simulink model "BrowarModel"  (R2024a)
settings: Solver=ode5  StartTime=0.0  StopTime=inf  FixedStep=0.1  RelTol=1e-3
undefined symbols (not defined in the file or in its folder): localhost, Matrikon, OI
libraries: opclib x24
(part 7 of 9)

== system BrowarModel/System dozowania drozdzy/System dozowania drozdzy/Zawor trojdrozny ==
  note: Zawor trojdrozny
  Sterowanie rusztem : Inport
  Przeplyw zasilanie : Inport  Port=2
  Dot Product : DotProduct  OutDataTypeStr=Inherit: Inherit via internal rule
  Relay : Relay  OffOutputValue=-1
  Transfer Fcn : TransferFcn  Denominator=[0.1 1]
  Przeplyw sterowanie : Outport
  wires:
  Transfer Fcn/1 -> Przeplyw sterowanie/1
  Dot Product/1 -> Transfer Fcn/1
  Przeplyw zasilanie/1 -> Dot Product/1
  Relay/1 -> Dot Product/2
  Sterowanie rusztem/1 -> Relay/1

== system BrowarModel/System dozowania drozdzy/WT805/Zaklocenia pomiarowe ==
  Product1 : Product  InputSameDT=on  RndMeth=Zero  SaturateOnIntegerOverflow=on  OutDataTypeStr=Inherit: Same as first input
  Product3 : Product  InputSameDT=on  RndMeth=Zero  SaturateOnIntegerOverflow=on  OutDataTypeStr=Inherit: Same as first input
  Random Number : RandomNumber  Variance=.04  Seed=4365624  SampleTime=0.1
  Transfer Fcn1 : TransferFcn  Denominator=[0.5 1]
  Transfer Fcn2 : TransferFcn  Denominator=[0.5 1]
  Zaklocenia pomiarowe : Constant  Value=ZakloceniaPom
  Out : Outport
  wires:
  Random Number/1 -> Product3/1
  Product3/1 -> Transfer Fcn1/1
  Transfer Fcn1/1 -> Transfer Fcn2/1
  Transfer Fcn2/1 -> Out/1
  Zaklocenia pomiarowe/1 -> Product1/2
  [ZaklPom] -> Product1/1
  Product1/1 -> Product3/2

== system BrowarModel/System dozowania drozdzy/XT804/Zaklocenia pomiarowe ==
  Product1 : Product  InputSameDT=on  RndMeth=Zero  SaturateOnIntegerOverflow=on  OutDataTypeStr=Inherit: Same as first input
  Product3 : Product  InputSameDT=on  RndMeth=Zero  SaturateOnIntegerOverflow=on  OutDataTypeStr=Inherit: Same as first input
  Random Number : RandomNumber  Variance=.5  Seed=4365624  SampleTime=0.1
  Transfer Fcn1 : TransferFcn  Denominator=[0.5 1]
  Transfer Fcn2 : TransferFcn  Denominator=[0.5 1]
  Zaklocenia pomiarowe : Constant  Value=ZakloceniaPom
  Out : Outport
  wires:
  Random Number/1 -> Product3/1
  Product3/1 -> Transfer Fcn1/1
  Transfer Fcn1/1 -> Transfer Fcn2/1
  Transfer Fcn2/1 -> Out/1
  Zaklocenia pomiarowe/1 -> Product1/2
  [ZaklPom] -> Product1/1
  Product1/1 -> Product3/2

== system BrowarModel/Kadz fermentacyjna/Kadz fermentacyjna/Kadz/Model akumulacji ciepla w zbiorniku z ciecza ==
  Objetosc cieczy w zbiorniku : Inport
  Strumien odplywu cieczy : Inport  Port=2
  Strumien doplywu cieczy : Inport  Port=3
  Strumien cieplna dostepny : Inport  Port=4
  Strumien cieplo traconego : Inport  Port=5
  Temperatura strumien doplywu cieczy : Inport  Port=6
  1/gestosc cieczy : Gain  Gain=1/1000
  Cieplo : Integrator  LimitOutput=on  LowerSaturationLimit=0
  Cieplo parowania : Constant  Value=2257000
  Cieplo strumienia cieczy doplywajacej : Subsystem
  Cieplo strumienia cieczy odplywajacej : Subsystem
  "Cieplo wlasciwe " : Constant  Value=4189.9
  Divide : Product  Inputs=/*
  Divide1 : Product  Inputs=*/
  Divide2 : Product  Inputs=*/
  "Dot " : DotProduct  OutDataTypeStr=Inherit: Inherit via internal rule
  Dot 1 : DotProduct  OutDataTypeStr=Inherit: Inherit via internal rule
  Gestosc cieczy : Gain  Gain=1000
  Saturation : Saturate  UpperLimit=inf  LowerLimit=0
  Sum{1..2,4..5} (4 alike) : Sum  Inputs=|+-
  Sum10 : Sum  Inputs=|++
  Sum3 : Sum  Inputs=|-+
  Sum7 : Sum  Inputs=|++
  Temperatura parowania : Constant  Value=100
  Zamiana C->K : Constant  Value=273.6
  Srumien cieczy odparowanej : Outport
  Srednia temperaturacie czy : Outport  Port=2
  Strumien ciepla odebrany : Outport  Port=3
  wires:
  Strumien cieplna dostepny/1 -> Strumien ciepla odebrany/1, Sum10/2  "J/s"
  Sum5/1 -> Sum4/1, Srednia temperaturacie czy/1
  Strumien doplywu cieczy/1 -> Cieplo strumienia cieczy doplywajacej/2(Strumien cieczy)  "m3/s"
  Zamiana C->K/1 -> Sum5/2
  "Cieplo wlasciwe "/1 -> Divide1/2, Dot 1/2  "J/(kg*K)"
  Cieplo strumienia cieczy doplywajacej/1(Strumien ciepla) -> Sum3/2  "J/s"
  Temperatura strumien doplywu cieczy/1 -> Cieplo strumienia cieczy doplywajacej/1(Temperatura strumienia cieczy)  "dec C"
  Divide1/1 -> Sum5/1, Cieplo strumienia cieczy odplywajacej/1(Temperatura strumienia cieczy)  "dec K"
  Divide/1 -> Divide1/1
  Cieplo/1 -> Divide/2  "J"
  Sum3/1 -> Sum1/1  "J/s"
  Strumien cieplo traconego/1 -> Sum1/2  "J/s"
  Sum1/1 -> Sum10/1  "J/s"
  Sum10/1 -> Sum2/1  "J/s"
  Temperatura parowania/1 -> Sum4/2  "dec C"
  Sum4/1 -> Saturation/1
  Saturation/1 -> Dot 1/1
  Dot 1/1 -> "Dot "/1
  "Dot "/1 -> Divide2/1, Sum2/2  "J/s"
  Sum2/1 -> Cieplo/1  "J/s"
  Cieplo strumienia cieczy odplywajacej/1(Strumien ciepla) -> Sum3/1  "J/s"
  1/gestosc cieczy/1 -> Sum7/2, Srumien cieczy odparowanej/1  "m3/s"
  Divide2/1 -> 1/gestosc cieczy/1  "kg/s"
  Cieplo parowania/1 -> Divide2/2  "J/kg"
  Objetosc cieczy w zbiorniku/1 -> Gestosc cieczy/1  "m3"
  Gestosc cieczy/1 -> "Dot "/2, Divide/1  "kg"
  Sum7/1 -> Cieplo strumienia cieczy odplywajacej/2(Strumien cieczy)
  Strumien odplywu cieczy/1 -> Sum7/1  "m3/s"

== system BrowarModel/Kadz fermentacyjna/Kadz fermentacyjna/Kadz/Model rozkladu temperatur ==
  note: Model rozkladu temperatur
  Poziom : Inport
  Srednia temperatura : Inport  Port=2
  Obroty mieszadla : Inport  Port=3
  " Dot 1" : DotProduct  OutDataTypeStr=Inherit: Inherit via internal rule
  " Dot 2" : DotProduct  OutDataTypeStr=Inherit: Inherit via internal rule
  " Dot 3" : DotProduct  OutDataTypeStr=Inherit: Inherit via internal rule
  Divide2 : Product  Inputs=/*
  Divide3 : Product  Inputs=/*
  Divide4 : Product  Inputs=/*
  Model rozkladu temperatur : Subsystem
  Pozycja sensor dolny : Constant  Value=0.5
  Pozycja sensor gorny : Constant  Value=2.5
  Pozycja sensor srodkowy : Constant  Value=1.5
  Sensor dolny niezanuzony : RelationalOperator  Operator=<  InputSameDT=off
  Sensor gorny niezanuzony : RelationalOperator  Operator=<  InputSameDT=off
  Sensor srodkowy niezanuzony : RelationalOperator  Operator=<  InputSameDT=off
  Sum13 : Sum  Inputs=|+-
  Sum14 : Sum  Inputs=|+-
  Sum15 : Sum  Inputs=|+-
  Switch : Switch  Threshold=0.5  SaturateOnIntegerOverflow=off  InputSameDT=off
  Switch1 : Switch  Threshold=0.5  SaturateOnIntegerOverflow=off  InputSameDT=off
  Switch2 : Switch  Threshold=0.5  SaturateOnIntegerOverflow=off  InputSameDT=off
  "Temperatura pokojowa (deg C) " : Constant  Value=22
  Temperatura lustra zbiornika : Outport
  Sensor temperatury gorny : Outport  Port=2
  Sensor temperatury srodkowy : Outport  Port=3
  Sensor temperatury dolny : Outport  Port=4
  Temperatura przy dnie zbiornika : Outport  Port=5
  wires:
  Model rozkladu temperatur/1(Temperatura przy powierzchni) -> Temperatura lustra zbiornika/1
  Poziom/1 -> Divide4/1, Divide3/1, Divide2/1, Sensor dolny niezanuzony/1, Sensor srodkowy niezanuzony/1, Sensor gorny niezanuzony/1, Model rozkladu temperatur/1(Poziom)  "m"
  Switch2/1 -> Sensor temperatury dolny/1
  Switch/1 -> Sensor temperatury gorny/1
  " Dot 3"/1 -> Sum15/2
  Divide2/1 -> " Dot 3"/2
  Divide3/1 -> " Dot 2"/2
  " Dot 2"/1 -> Sum14/2
  " Dot 1"/1 -> Sum13/2
  Divide4/1 -> " Dot 1"/2
  Model rozkladu temperatur/2(Temperatura przy dnie) -> Sum15/1, Sum14/1, Sum13/1, Temperatura przy dnie zbiornika/1
  Sum15/1 -> Switch2/3
  Sum14/1 -> Switch1/3
  Sum13/1 -> Switch/3
  Switch1/1 -> Sensor temperatury srodkowy/1
  Sensor dolny niezanuzony/1 -> Switch2/2
  Sensor srodkowy niezanuzony/1 -> Switch1/2
  Sensor gorny niezanuzony/1 -> Switch/2
  Pozycja sensor dolny/1 -> Divide2/2, Sensor dolny niezanuzony/2
  Pozycja sensor srodkowy/1 -> Divide3/2, Sensor srodkowy niezanuzony/2
  Pozycja sensor gorny/1 -> Divide4/2, Sensor gorny niezanuzony/2
  "Temperatura pokojowa (deg C) "/1 -> Switch2/1, Switch1/1, Switch/1, Model rozkladu temperatur/2(Temperatura otoczenia)
  Model rozkladu temperatur/3(Gradient temperatury) -> " Dot 1"/1, " Dot 2"/1, " Dot 3"/1
  Srednia temperatura/1 -> Model rozkladu temperatur/3(Srednia temperatura)  "decC"
  Obroty mieszadla/1 -> Model rozkladu temperatur/4(Obroty mieszadla)  "obr/min"

== system BrowarModel/Kadz fermentacyjna/Kadz fermentacyjna/Kadz/Model utratu ciepla ==
  note: Model utraty ciepla
  Poziom : Inport
  Pole podstawy zbiornika : Inport  Port=2
  Srednia temperatura : Inport  Port=3
  Temperatura lustra : Inport  Port=4
  Cieplo tracone przez pow. gorna : DotProduct  OutDataTypeStr=Inherit: Inherit via internal rule
  Cieplo tracone przez scianki : DotProduct  OutDataTypeStr=Inherit: Inherit via internal rule
  Pow ->obwod : Fcn  Expr=2*3.14*sqrt(u(1)/3.14)
  Pow styku scian bocznych : DotProduct  OutDataTypeStr=Inherit: Inherit via internal rule
  Saturation : Saturate  UpperLimit=inf  LowerLimit=0
  Sum11 : Sum  Inputs=|-+
  Sum12 : Sum  Inputs=|-+
  Sum2 : Sum
  "Temperatura pokojowa (deg C)  " : Constant  Value=22
  Wspolczynnik przenikania ciepla : Gain  Gain=950
  Wspolczynnik przenikania ciepla scian : Gain  Gain=450
  Strumien ciepla : Outport
  wires:
  Temperatura lustra/1 -> Sum12/2  "dec C"
  Sum2/1 -> Saturation/1
  Srednia temperatura/1 -> Sum11/2  "dec C"
  Pole podstawy zbiornika/1 -> Wspolczynnik przenikania ciepla/1, Pow ->obwod/1
  Poziom/1 -> Pow styku scian bocznych/1
  Sum11/1 -> Cieplo tracone przez scianki/2
  "Temperatura pokojowa (deg C)  "/1 -> Sum12/1, Sum11/1
  Cieplo tracone przez pow. gorna/1 -> Sum2/2
  Cieplo tracone przez scianki/1 -> Sum2/1
  Wspolczynnik przenikania ciepla scian/1 -> Cieplo tracone przez scianki/1
  Pow styku scian bocznych/1 -> Wspolczynnik przenikania ciepla scian/1  "m2"
  Pow ->obwod/1 -> Pow styku scian bocznych/2
  Sum12/1 -> Cieplo tracone przez pow. gorna/1
  Wspolczynnik przenikania ciepla/1 -> Cieplo tracone przez pow. gorna/2
  Saturation/1 -> Strumien ciepla/1  "J/s"

== system BrowarModel/Kadz fermentacyjna/Kadz fermentacyjna/Kadz/Poziom zbiornika ==
  note: Poziom zbiornika
  Objetosc : Inport
  Powierzchnia dna : Inport  Port=2
  1/powierzchnia : Product  Inputs=*/
  Pozycja sensora max (2.8 m) : Constant  Value=2.8
  Pozycja sensora min (0.2 m) : Constant  Value=.2
  Sensor max : RelationalOperator  InputSameDT=off
  Sensor min : RelationalOperator  InputSameDT=off
  Poziom  wysoki : Outport
  Poziom niski : Outport  Port=2
  Poziom : Outport  Port=3
  wires:
  Objetosc/1 -> 1/powierzchnia/1  "m3"
  Powierzchnia dna/1 -> 1/powierzchnia/2  "m2"
  Sensor min/1 -> Poziom niski/1
  Sensor max/1 -> Poziom  wysoki/1
  Pozycja sensora min (0.2 m)/1 -> Sensor min/2
  Pozycja sensora max (2.8 m)/1 -> Sensor max/2
  1/powierzchnia/1 -> Poziom/1, Sensor max/1, Sensor min/1  "m"

== system BrowarModel/Kadz fermentacyjna/Kadz fermentacyjna/Model ogrzewacza/Zaklocenia ==
  note: Zaklocenia procesowe
  In : Inport
  Product3 : Product  InputSameDT=on  RndMeth=Zero  SaturateOnIntegerOverflow=on  OutDataTypeStr=Inherit: Same as first input
  Product4 : Product  InputSameDT=on  RndMeth=Zero  SaturateOnIntegerOverflow=on  OutDataTypeStr=Inherit: Same as first input
  Random Number : RandomNumber  Seed=4365624  SampleTime=0.1
  Transfer Fcn1 : TransferFcn  Denominator=[10 1]
  Transfer Fcn2 : TransferFcn  Denominator=[10 1]
  Transfer Fcn3 : TransferFcn  Denominator=[10 1]
  Out : Outport
  wires:
  [ZaklProc] -> Product3/2
  Random Number/1 -> Product3/1
  Product3/1 -> Transfer Fcn1/1
  Transfer Fcn1/1 -> Transfer Fcn2/1
  In/1 -> Product4/1
  Product4/1 -> Out/1
  Transfer Fcn2/1 -> Transfer Fcn3/1
  Transfer Fcn3/1 -> Product4/2

== system BrowarModel/Kadz fermentacyjna/Kadz fermentacyjna/Odplyw z kadzi/Silnik elektryczny ==
  note: Silnik elektryczny
  note: Uszkodzenie silnika
  Zalaczenie : Inport
  Zadane obroty : Inport  Port=2
  Obciazenie zew : Inport  Port=3
  Uszkodzenie : Inport  Port=4
  Abs : Abs  SaturateOnIntegerOverflow=off
  Add : Sum
  Add1 : Sum  Inputs=+-
  Const : Constant
  Gain : Gain
  "Hz -> obr/min" : Gain  Gain=60/2
  Inercja mechaniczna : TransferFcn  Denominator=[1 1]
  Poslizg : DotProduct  OutDataTypeStr=Inherit: Inherit via internal rule
  Poslizg jalowy : Constant  Value=0.04
  Poslizg od obciazenia : Gain  Gain=0.05
  Prad jalowy : Gain  Gain=0.5
  Prad nominalny (10A) : Constant  Value=10
  Relay : Relay  OnOutputValue=0  OffOutputValue=1
  Saturation [0,1] : Saturate  UpperLimit=1  LowerLimit=0
  "Saturation [0,1] " : Saturate  UpperLimit=1  LowerLimit=0
  Stan : Subsystem
  Sterowanie : Subsystem
  Sterownik : Subsystem
  Sum : Sum  Inputs=|+-
  Sum1 : Sum  Inputs=|++
  Sum2 : Sum  Inputs=|+-
  Sum3 : Sum  Inputs=|++
  Wplyw uszkodzenia : DotProduct  OutDataTypeStr=Inherit: Inherit via internal rule
  Wplyw obciazenia : DotProduct  OutDataTypeStr=Inherit: Inherit via internal rule
  Wplyw obrotow : DotProduct  OutDataTypeStr=Inherit: Inherit via internal rule
  Zaklocenia : Subsystem
  Zalaczony : DotProduct  OutDataTypeStr=Inherit: Inherit via internal rule
  "obr/min -> FS  " : Gain  Gain=1/1500
  "obr/min -> Hz" : Gain  Gain=1/60*2
  Obroty : Outport
  Prad : Outport  Port=2
  Idle : Outport  Port=3
  Running : Outport  Port=4
  Alarm : Outport  Port=5
  wires:
  Inercja mechaniczna/1 -> Obroty/1, Poslizg/1, Add1/2, "obr/min -> Hz"/1
  Sum/1 -> Inercja mechaniczna/1
  "Hz -> obr/min"/1 -> Sum2/1, Zaklocenia/1(In)  "[obr/min]"
  Poslizg/1 -> Sum/2
  Sum3/1 -> Poslizg/2
  Poslizg od obciazenia/1 -> Sum3/1
  Obciazenie zew/1 -> Saturation [0,1]/1  "FS"
  Poslizg jalowy/1 -> Sum3/2
  Prad nominalny (10A)/1 -> Prad jalowy/1  "A"
  Prad jalowy/1 -> Sum1/2, Wplyw obciazenia/2
  Wplyw obciazenia/1 -> Sum1/1
  Abs/1 -> Wplyw obciazenia/1  "FS"
  Const/1 -> Wplyw obrotow/1
  "obr/min -> Hz"/1 -> Sterownik/1(PV)
  Saturation [0,1]/1 -> Add/2
  Add/1 -> Poslizg od obciazenia/1, Abs/1  "FS"
  Add1/1 -> "obr/min -> FS  "/1
  "obr/min -> FS  "/1 -> Gain/1
  "Saturation [0,1] "/1 -> Add/1
  Zalaczenie/1 -> Sterowanie/2(Zalaczenie), Stan/1(Zalaczony)
  Sterowanie/1(Sterowanie) -> Sterownik/2(SP)
  Gain/1 -> "Saturation [0,1] "/1
  Uszkodzenie/1 -> Relay/1
  Sterownik/1(CV) -> Wplyw uszkodzenia/1
  Relay/1 -> Wplyw uszkodzenia/2, Stan/2(Zdatny)
  Wplyw uszkodzenia/1 -> "Hz -> obr/min"/1
  Wplyw obrotow/1 -> Prad/1  "A"
  Sum1/1 -> Zalaczony/1  "A"
  Zalaczony/1 -> Wplyw obrotow/2
  Zadane obroty/1 -> Sterowanie/1(Zadane obroty)
  Stan/1(Idle) -> Idle/1
  Stan/2(Running) -> Running/1, Zalaczony/2
  Stan/3(Alarm) -> Alarm/1
  Sum2/1 -> Add1/1, Sum/1
  Zaklocenia/1(Out) -> Sum2/2

== system BrowarModel/Kadz fermentacyjna/Kadz fermentacyjna/Odplyw z kadzi/Zawor dyskretny ==
  note: Model zaworu dyskretnego
  Sterowanie : Inport
  Cisnienie : Inport  Port=2
  Przeciek : Inport  Port=3
  Dlawienie : Inport  Port=4
  Const : Constant  Value=100
  GUIMon : Gain
  Gain : Gain  Gain=(0.15/sqrt(300))/100
  Gain1 : Gain  Gain=1/100
  Integer Delay : Delay  DelayLength=15
  Math Function : Math  Operator=sqrt  SignedPower=on
  Product : Product  RndMeth=Zero
  Product1 : Product  RndMeth=Zero
  Relay : Relay  OnOutputValue=100
  Sat (0-100) : Saturate  UpperLimit=100  LowerLimit=0
  Sat dlawienia (0-100) : Saturate  UpperLimit=100  LowerLimit=0
  Sat przecieku (0-100) : Saturate  UpperLimit=100  LowerLimit=0
  Sum3 : Sum  Inputs=|+-
  Sum4 : Sum  Inputs=|++
  Transfer Fcn : TransferFcn  Denominator=[0.2 1]
  Przeplyw : Outport
  wires:
  Const/1 -> Sum3/1
  Sat dlawienia (0-100)/1 -> Sum3/2
  Sum3/1 -> Gain1/1
  Sat (0-100)/1 -> Product/1
  Sum4/1 -> Sat (0-100)/1
  Relay/1 -> GUIMon/1
  Sat przecieku (0-100)/1 -> Sum4/2
  Sterowanie/1 -> Relay/1
  Product/1 -> Product1/2  "[0,1]"
  Przeciek/1 -> Sat przecieku (0-100)/1
  Dlawienie/1 -> Sat dlawienia (0-100)/1
  Product1/1 -> Transfer Fcn/1
  Gain/1 -> Integer Delay/1  "m3/s"
  Cisnienie/1 -> Math Function/1  "kPa"
  Math Function/1 -> Product1/1
  Transfer Fcn/1 -> Gain/1
  Integer Delay/1 -> Przeplyw/1
  GUIMon/1 -> Sum4/1
  Gain1/1 -> Product/2

== system BrowarModel/Kadz fermentacyjna/Kadz fermentacyjna/Silnik elektryczny/Stan ==
  Zalaczony : Inport
  Zdatny : Inport  Port=2
  Add : Sum  Inputs=+++
  Alarm1 : Logic  Operator=NOT  AllPortsSameDT=off
  Alarm2 : Gain  Gain=3
  Display : Display
  GUIMon : Gain
  Idle1 : Logic  AllPortsSameDT=off
  Idle2 : Logic  Operator=NOT  AllPortsSameDT=off
  Idle3 : Gain
  Running1 : Logic  AllPortsSameDT=off
  Running2 : Gain  Gain=2
  Idle : Outport
  Running : Outport  Port=2
  Alarm : Outport  Port=3
  wires:
  GUIMon/1 -> Display/1
  Add/1 -> GUIMon/1
  Alarm2/1 -> Add/3
  Running2/1 -> Add/2
  Idle3/1 -> Add/1
  Idle2/1 -> Idle1/1
  Alarm1/1 -> Alarm2/1, Alarm/1
  Zdatny/1 -> Idle1/2, Running1/2, Alarm1/1
  Zalaczony/1 -> Idle2/1, Running1/1
  Idle1/1 -> Idle3/1, Idle/1
  Running1/1 -> Running2/1, Running/1

== system BrowarModel/Kadz fermentacyjna/Kadz fermentacyjna/Silnik elektryczny/Sterowanie ==
  note: Sterowanie silnika elektrycznego
  Zadane obroty : Inport
  Zalaczenie : Inport  Port=2
  Hz : Gain  Gain=45/100
  Min sterowanie : Constant  Value=5
  Relay : Relay
  Saturation [0,100] : Saturate  UpperLimit=100  LowerLimit=0
  "Sterowanie " : DotProduct  OutDataTypeStr=Inherit: Inherit via internal rule
  Sum2 : Sum  Inputs=|++
  Sterowanie : Outport
  wires:
  Zadane obroty/1 -> Saturation [0,100]/1  "[0,100]"
  "Sterowanie "/1 -> Sterowanie/1  "Hz"
  Zalaczenie/1 -> Relay/1  "{0,1}"
  Sum2/1 -> "Sterowanie "/2
  Min sterowanie/1 -> Sum2/2  "Hz"
  Hz/1 -> Sum2/1  "Hz"
  Saturation [0,100]/1 -> Hz/1
  Relay/1 -> "Sterowanie "/1  "{0,1}"

== system BrowarModel/Kadz fermentacyjna/Kadz fermentacyjna/Silnik elektryczny/Sterownik ==
  PV : Inport
  SP : Inport  Port=2
  Integrator : Integrator  LimitOutput=on  UpperSaturationLimit=50  LowerSaturationLimit=0
  K : Gain
  Saturation [0,50] : Saturate  UpperLimit=50  LowerLimit=0
  Sum2 : Sum  Inputs=|+-
  Sum3 : Sum  Inputs=|++
  Ti : Gain
  CV : Outport
  wires:
  Saturation [0,50]/1 -> CV/1
  Sum3/1 -> Saturation [0,50]/1
  SP/1 -> Sum2/1
  PV/1 -> Sum2/2
  Ti/1 -> Integrator/1
  K/1 -> Sum3/2, Ti/1
  Integrator/1 -> Sum3/1
  Sum2/1 -> K/1

== system BrowarModel/Kadz fermentacyjna/Kadz fermentacyjna/Silnik elektryczny/Zaklocenia ==
  note: Zaklocenia procesowe
  In : Inport
  Product3 : Product  InputSameDT=on  RndMeth=Zero  SaturateOnIntegerOverflow=on  OutDataTypeStr=Inherit: Same as first input
  Product4 : Product  InputSameDT=on  RndMeth=Zero  SaturateOnIntegerOverflow=on  OutDataTypeStr=Inherit: Same as first input
  Random Number : RandomNumber  Variance=0.05  Seed=4365624  SampleTime=0.1
  Transfer Fcn1 : TransferFcn  Denominator=[1 1]
  Transfer Fcn2 : TransferFcn  Denominator=[1 1]
  Transfer Fcn3 : TransferFcn  Denominator=[1 1]
  Out : Outport
  wires:
  Transfer Fcn3/1 -> Product4/2
  Transfer Fcn2/1 -> Transfer Fcn3/1
  Product4/1 -> Out/1
  In/1 -> Product4/1
  Transfer Fcn1/1 -> Transfer Fcn2/1
  Product3/1 -> Transfer Fcn1/1
  Random Number/1 -> Product3/1
  [ZaklProc] -> Product3/2

== system BrowarModel/Kadz filtracji/Kadz filtracji/Doplyw kadzi/Silnik elektryczny ==
  note: Silnik elektryczny
  note: Uszkodzenie silnika
  Zalaczenie : Inport
  Zadane obroty : Inport  Port=2
  Obciazenie zew : Inport  Port=3
  Uszkodzenie : Inport  Port=4
  Abs : Abs  SaturateOnIntegerOverflow=off
  Add : Sum
  Add1 : Sum  Inputs=+-
  Const : Constant
  Gain : Gain
  "Hz -> obr/min" : Gain  Gain=60/2
  Inercja mechaniczna : TransferFcn  Denominator=[1 1]
  Poslizg : DotProduct  OutDataTypeStr=Inherit: Inherit via internal rule
  Poslizg jalowy : Constant  Value=0.04
  Poslizg od obciazenia : Gain  Gain=0.05
  Prad jalowy : Gain  Gain=0.5
  Prad nominalny (10A) : Constant  Value=10
  Relay : Relay  OnOutputValue=0  OffOutputValue=1
  Saturation [0,1] : Saturate  UpperLimit=1  LowerLimit=0
  "Saturation [0,1] " : Saturate  UpperLimit=1  LowerLimit=0
  Stan : Subsystem
  Sterowanie : Subsystem
  Sterownik : Subsystem
  Sum : Sum  Inputs=|+-
  Sum1 : Sum  Inputs=|++
  Sum2 : Sum  Inputs=|+-
  Sum3 : Sum  Inputs=|++
  Wplyw uszkodzenia : DotProduct  OutDataTypeStr=Inherit: Inherit via internal rule
  Wplyw obciazenia : DotProduct  OutDataTypeStr=Inherit: Inherit via internal rule
  Wplyw obrotow : DotProduct  OutDataTypeStr=Inherit: Inherit via internal rule
  Zaklocenia : Subsystem
  Zalaczony : DotProduct  OutDataTypeStr=Inherit: Inherit via internal rule
  "obr/min -> FS  " : Gain  Gain=1/1500
  "obr/min -> Hz" : Gain  Gain=1/60*2
  Obroty : Outport
  Prad : Outport  Port=2
  Idle : Outport  Port=3
  Running : Outport  Port=4
  Alarm : Outport  Port=5
  wires:
  Inercja mechaniczna/1 -> Obroty/1, Poslizg/1, Add1/2, "obr/min -> Hz"/1
  Sum/1 -> Inercja mechaniczna/1
  "Hz -> obr/min"/1 -> Sum2/1, Zaklocenia/1(In)  "[obr/min]"
  Poslizg/1 -> Sum/2
  Sum3/1 -> Poslizg/2
  Poslizg od obciazenia/1 -> Sum3/1
  Obciazenie zew/1 -> Saturation [0,1]/1  "FS"
  Poslizg jalowy/1 -> Sum3/2
  Prad nominalny (10A)/1 -> Prad jalowy/1  "A"
  Prad jalowy/1 -> Sum1/2, Wplyw obciazenia/2
  Wplyw obciazenia/1 -> Sum1/1
  Abs/1 -> Wplyw obciazenia/1  "FS"
  Const/1 -> Wplyw obrotow/1
  "obr/min -> Hz"/1 -> Sterownik/1(PV)
  Saturation [0,1]/1 -> Add/2
  Add/1 -> Poslizg od obciazenia/1, Abs/1  "FS"
  Add1/1 -> "obr/min -> FS  "/1
  "obr/min -> FS  "/1 -> Gain/1
  "Saturation [0,1] "/1 -> Add/1
  Zalaczenie/1 -> Sterowanie/2(Zalaczenie), Stan/1(Zalaczony)
  Sterowanie/1(Sterowanie) -> Sterownik/2(SP)
  Gain/1 -> "Saturation [0,1] "/1
  Uszkodzenie/1 -> Relay/1
  Sterownik/1(CV) -> Wplyw uszkodzenia/1
  Relay/1 -> Wplyw uszkodzenia/2, Stan/2(Zdatny)
  Wplyw uszkodzenia/1 -> "Hz -> obr/min"/1
  Wplyw obrotow/1 -> Prad/1  "A"
  Sum1/1 -> Zalaczony/1  "A"
  Zalaczony/1 -> Wplyw obrotow/2
  Zadane obroty/1 -> Sterowanie/1(Zadane obroty)
  Stan/1(Idle) -> Idle/1
  Stan/2(Running) -> Running/1, Zalaczony/2
  Stan/3(Alarm) -> Alarm/1
  Sum2/1 -> Add1/1, Sum/1
  Zaklocenia/1(Out) -> Sum2/2

== system BrowarModel/Kadz filtracji/Kadz filtracji/Doplyw kadzi/Zawor dyskretny ==
  note: Model zaworu dyskretnego
  Sterowanie : Inport
  Cisnienie : Inport  Port=2
  Przeciek : Inport  Port=3
  Dlawienie : Inport  Port=4
  Const : Constant  Value=100
  Dead Zone : DeadZone  LowerValue=-inf  UpperValue=0.001
  GUIMon : Gain
  Gain : Gain  Gain=(0.15/sqrt(300))/100
  Gain1 : Gain  Gain=1/100
  Integer Delay : Delay  DelayLength=15
  Math Function : Math  Operator=sqrt  SignedPower=on
  Product : Product  RndMeth=Zero
  Product1 : Product  RndMeth=Zero
  Relay : Relay  OnOutputValue=100
  Sat (0-100) : Saturate  UpperLimit=100  LowerLimit=0
  Sat dlawienia (0-100) : Saturate  UpperLimit=100  LowerLimit=0
  Sat przecieku (0-100) : Saturate  UpperLimit=100  LowerLimit=0
  Sum3 : Sum  Inputs=|+-
  Sum4 : Sum  Inputs=|++
  Transfer Fcn : TransferFcn  Denominator=[0.2 1]
  Przeplyw : Outport
  wires:
  Const/1 -> Sum3/1
  Sat dlawienia (0-100)/1 -> Sum3/2
  Sum3/1 -> Gain1/1
  Sat (0-100)/1 -> Product/1
  Sum4/1 -> Sat (0-100)/1
  Relay/1 -> GUIMon/1
  Sat przecieku (0-100)/1 -> Sum4/2
  Sterowanie/1 -> Relay/1
  Product/1 -> Product1/2  "[0,1]"
  Przeciek/1 -> Sat przecieku (0-100)/1
  Dlawienie/1 -> Sat dlawienia (0-100)/1
  Product1/1 -> Transfer Fcn/1
  Gain/1 -> Integer Delay/1  "m3/s"
  Cisnienie/1 -> Math Function/1  "kPa"
  Math Function/1 -> Product1/1
  Transfer Fcn/1 -> Gain/1
  Integer Delay/1 -> Dead Zone/1
  GUIMon/1 -> Sum4/1
  Gain1/1 -> Product/2
  Dead Zone/1 -> Przeplyw/1

== system BrowarModel/Kadz filtracji/Kadz filtracji/Odplyw + cyrkulacja/Silnik elektryczny ==
  note: Silnik elektryczny
  note: Uszkodzenie silnika
  Zalaczenie : Inport
  Zadane obroty : Inport  Port=2
  Obciazenie zew : Inport  Port=3
  Uszkodzenie : Inport  Port=4
  Abs : Abs  SaturateOnIntegerOverflow=off
  Add : Sum
  Add1 : Sum  Inputs=+-
  Const : Constant
  Gain : Gain
  "Hz -> obr/min" : Gain  Gain=60/2
  Inercja mechaniczna : TransferFcn  Denominator=[1 1]
  Poslizg : DotProduct  OutDataTypeStr=Inherit: Inherit via internal rule
  Poslizg jalowy : Constant  Value=0.04
  Poslizg od obciazenia : Gain  Gain=0.05
  Prad jalowy : Gain  Gain=0.5
  Prad nominalny (10A) : Constant  Value=10
  Relay : Relay  OnOutputValue=0  OffOutputValue=1
  Saturation [0,1] : Saturate  UpperLimit=1  LowerLimit=0
  "Saturation [0,1] " : Saturate  UpperLimit=1  LowerLimit=0
  Stan : Subsystem
  Sterowanie : Subsystem
  Sterownik : Subsystem
  Sum : Sum  Inputs=|+-
  Sum1 : Sum  Inputs=|++
  Sum2 : Sum  Inputs=|+-
  Sum3 : Sum  Inputs=|++
  Wplyw uszkodzenia : DotProduct  OutDataTypeStr=Inherit: Inherit via internal rule
  Wplyw obciazenia : DotProduct  OutDataTypeStr=Inherit: Inherit via internal rule
  Wplyw obrotow : DotProduct  OutDataTypeStr=Inherit: Inherit via internal rule
  Zaklocenia : Subsystem
  Zalaczony : DotProduct  OutDataTypeStr=Inherit: Inherit via internal rule
  "obr/min -> FS  " : Gain  Gain=1/1500
  "obr/min -> Hz" : Gain  Gain=1/60*2
  Obroty : Outport
  Prad : Outport  Port=2
  Idle : Outport  Port=3
  Running : Outport  Port=4
  Alarm : Outport  Port=5
  wires:
  Inercja mechaniczna/1 -> Obroty/1, Poslizg/1, Add1/2, "obr/min -> Hz"/1
  Sum/1 -> Inercja mechaniczna/1
  "Hz -> obr/min"/1 -> Sum2/1, Zaklocenia/1(In)  "[obr/min]"
  Poslizg/1 -> Sum/2
  Sum3/1 -> Poslizg/2
  Poslizg od obciazenia/1 -> Sum3/1
  Obciazenie zew/1 -> Saturation [0,1]/1  "FS"
  Poslizg jalowy/1 -> Sum3/2
  Prad nominalny (10A)/1 -> Prad jalowy/1  "A"
  Prad jalowy/1 -> Sum1/2, Wplyw obciazenia/2
  Wplyw obciazenia/1 -> Sum1/1
  Abs/1 -> Wplyw obciazenia/1  "FS"
  Const/1 -> Wplyw obrotow/1
  "obr/min -> Hz"/1 -> Sterownik/1(PV)
  Saturation [0,1]/1 -> Add/2
  Add/1 -> Poslizg od obciazenia/1, Abs/1  "FS"
  Add1/1 -> "obr/min -> FS  "/1
  "obr/min -> FS  "/1 -> Gain/1
  "Saturation [0,1] "/1 -> Add/1
  Zalaczenie/1 -> Sterowanie/2(Zalaczenie), Stan/1(Zalaczony)
  Sterowanie/1(Sterowanie) -> Sterownik/2(SP)
  Gain/1 -> "Saturation [0,1] "/1
  Uszkodzenie/1 -> Relay/1
  Sterownik/1(CV) -> Wplyw uszkodzenia/1
  Relay/1 -> Wplyw uszkodzenia/2, Stan/2(Zdatny)
  Wplyw uszkodzenia/1 -> "Hz -> obr/min"/1
  Wplyw obrotow/1 -> Prad/1  "A"
  Sum1/1 -> Zalaczony/1  "A"
  Zalaczony/1 -> Wplyw obrotow/2
  Zadane obroty/1 -> Sterowanie/1(Zadane obroty)
  Stan/1(Idle) -> Idle/1
  Stan/2(Running) -> Running/1, Zalaczony/2
  Stan/3(Alarm) -> Alarm/1
  Sum2/1 -> Add1/1, Sum/1
  Zaklocenia/1(Out) -> Sum2/2

== system BrowarModel/Kadz filtracji/Kadz filtracji/Odplyw + cyrkulacja/Zawor dyskretny - powrot ==
  note: Model zaworu dyskretnego
  Sterowanie : Inport
  Cisnienie : Inport  Port=2
  Przeciek : Inport  Port=3
  Dlawienie : Inport  Port=4
  Const : Constant  Value=100
  Dead Zone : DeadZone  LowerValue=-inf  UpperValue=0.002
  GUIMon : Gain
  Gain : Gain  Gain=(0.15/sqrt(300))/100
  Gain1 : Gain  Gain=1/100
  Integer Delay : Delay  DelayLength=15
  Math Function : Math  Operator=sqrt  SignedPower=on
  Product : Product  RndMeth=Zero
  Product1 : Product  RndMeth=Zero
  Relay : Relay  OnOutputValue=100
  Sat (0-100) : Saturate  UpperLimit=100  LowerLimit=0
  Sat dlawienia (0-100) : Saturate  UpperLimit=100  LowerLimit=0
  Sat przecieku (0-100) : Saturate  UpperLimit=100  LowerLimit=0
  Sum3 : Sum  Inputs=|+-
  Sum4 : Sum  Inputs=|++
  Transfer Fcn : TransferFcn  Denominator=[0.2 1]
  Przeplyw : Outport
  wires:
  Const/1 -> Sum3/1
  Sat dlawienia (0-100)/1 -> Sum3/2
  Sum3/1 -> Gain1/1
  Sat (0-100)/1 -> Product/1
  Sum4/1 -> Sat (0-100)/1
  Relay/1 -> GUIMon/1
  Sat przecieku (0-100)/1 -> Sum4/2
  Sterowanie/1 -> Relay/1
  Product/1 -> Product1/2  "[0,1]"
  Przeciek/1 -> Sat przecieku (0-100)/1
  Dlawienie/1 -> Sat dlawienia (0-100)/1
  Product1/1 -> Gain/1
  Gain/1 -> Transfer Fcn/1  "m3/s"
  Cisnienie/1 -> Math Function/1  "kPa"
  Math Function/1 -> Product1/1
  Transfer Fcn/1 -> Integer Delay/1
  Integer Delay/1 -> Dead Zone/1
  GUIMon/1 -> Sum4/1
  Gain1/1 -> Product/2
  Dead Zone/1 -> Przeplyw/1

== system BrowarModel/Kadz filtracji/Kadz filtracji/Odplyw + cyrkulacja/Zawor dyskretny - spust ==
  note: Model zaworu dyskretnego
  Sterowanie : Inport
  Cisnienie : Inport  Port=2
  Przeciek : Inport  Port=3
  Dlawienie : Inport  Port=4
  Const : Constant  Value=100
  Dead Zone : DeadZone  LowerValue=-inf  UpperValue=0.002
  GUIMon : Gain
  Gain : Gain  Gain=(0.15/sqrt(300))/100
  Gain1 : Gain  Gain=1/100
  Integer Delay : Delay  DelayLength=15
  Math Function : Math  Operator=sqrt  SignedPower=on
  Product : Product  RndMeth=Zero
  Product1 : Product  RndMeth=Zero
  Relay : Relay  OnOutputValue=100
  Sat (0-100) : Saturate  UpperLimit=100  LowerLimit=0
  Sat dlawienia (0-100) : Saturate  UpperLimit=100  LowerLimit=0
  Sat przecieku (0-100) : Saturate  UpperLimit=100  LowerLimit=0
  Sum3 : Sum  Inputs=|+-
  Sum4 : Sum  Inputs=|++
  Transfer Fcn : TransferFcn  Denominator=[0.2 1]
  Przeplyw : Outport
  wires:
  Math Function/1 -> Product1/1
  Cisnienie/1 -> Math Function/1  "kPa"
  Gain/1 -> Transfer Fcn/1  "m3/s"
  Product1/1 -> Gain/1
  Dlawienie/1 -> Sat dlawienia (0-100)/1
  Przeciek/1 -> Sat przecieku (0-100)/1
  Product/1 -> Product1/2  "[0,100]"
  Sterowanie/1 -> Relay/1
  Sat przecieku (0-100)/1 -> Sum4/2
  Relay/1 -> GUIMon/1
  Sum4/1 -> Sat (0-100)/1
  Sat (0-100)/1 -> Product/1
  Sum3/1 -> Gain1/1
  Sat dlawienia (0-100)/1 -> Sum3/2
  Const/1 -> Sum3/1
  Transfer Fcn/1 -> Integer Delay/1
  Integer Delay/1 -> Dead Zone/1
  GUIMon/1 -> Sum4/1
  Gain1/1 -> Product/2
  Dead Zone/1 -> Przeplyw/1

== system BrowarModel/Kadz filtracji/Kadz filtracji/Zawor doplywu wody/Zaklocenia ==
  note: Zaklocenia procesowe
  In : Inport
  Product3 : Product  InputSameDT=on  RndMeth=Zero  SaturateOnIntegerOverflow=on  OutDataTypeStr=Inherit: Same as first input
  Product4 : Product  InputSameDT=on  RndMeth=Zero  SaturateOnIntegerOverflow=on  OutDataTypeStr=Inherit: Same as first input
  Random Number : RandomNumber  Variance=0.01  Seed=4365624  SampleTime=0.1
  Transfer Fcn1 : TransferFcn  Denominator=[0.1 1]
  Out : Outport
  wires:
  [ZaklProc] -> Product3/2
  Random Number/1 -> Product3/1
  Product3/1 -> Transfer Fcn1/1
  Transfer Fcn1/1 -> Product4/2
  In/1 -> Product4/1
  Product4/1 -> Out/1

== system BrowarModel/Kadz filtracji/Kadz filtracji/Zbiornik dolny/Model akumulacji ciepla w zbiorniku ==
  note: Model akumulacji ciepla w zbiorniku
  Objetosc cieczy w zbiorniku : Inport
  Przepelnienie : Inport  Port=2
  Strumien brzeczki : Inport  Port=3
  Strumien odplywu cieczy : Inport  Port=4
  Temperatura strumien doplywu brzeczki : Inport  Port=5
  Strumien ciepla traconego : Inport  Port=6
  Cieplo : Integrator  InitialCondition=1238534.44  LimitOutput=on  LowerSaturationLimit=0
  Cieplo strumienia cieczy odplywajacej : Subsystem
  Cieplo strumienia doplywajacego : Subsystem
  "Cieplo wlasciwe " : Constant  Value=4189.9
  Divide : Product  Inputs=/*
  Divide1 : Product  Inputs=*/
  Gestosc cieczy : Gain  Gain=1000
  Sum1 : Sum  Inputs=|+-
  Sum3 : Sum  Inputs=|-+
  Sum5 : Sum  Inputs=|+-
  Switch : Switch  Threshold=0.5  SaturateOnIntegerOverflow=off  InputSameDT=off
  Switch1 : Switch  Threshold=-0.5  SaturateOnIntegerOverflow=off  InputSameDT=off
  Zamiana C->K : Constant  Value=273.6
  Zero : Constant  Value=0
  Temperatura : Outport
  wires:
  Strumien odplywu cieczy/1 -> Cieplo strumienia cieczy odplywajacej/2(Strumien cieczy)  "m3/s"
  Gestosc cieczy/1 -> Divide/1  "kg"
  Objetosc cieczy w zbiorniku/1 -> Gestosc cieczy/1  "m3"
  Cieplo/1 -> Divide/2  "J"
  Divide/1 -> Divide1/1
  Divide1/1 -> Cieplo strumienia cieczy odplywajacej/1(Temperatura strumienia cieczy), Sum5/1  "dec K"
  "Cieplo wlasciwe "/1 -> Divide1/2  "J/(kg*K)"
  Zamiana C->K/1 -> Sum5/2
  Sum5/1 -> Temperatura/1
  Przepelnienie/1 -> Switch/2, Switch1/2
  Cieplo strumienia doplywajacego/1(Strumien ciepla) -> Switch/3  "J/s"
  Switch/1 -> Sum3/2
  Cieplo strumienia cieczy odplywajacej/1(Strumien ciepla) -> Switch/1, Switch1/1  "J/s"
  Temperatura strumien doplywu brzeczki/1 -> Cieplo strumienia doplywajacego/1(Temperatura strumienia brzeczki)
  Strumien brzeczki/1 -> Cieplo strumienia doplywajacego/2(Strumien brzeczki)
  Switch1/1 -> Sum3/1
  Zero/1 -> Switch1/3
  Sum3/1 -> Sum1/1  "J/s"
  Sum1/1 -> Cieplo/1
  Strumien ciepla traconego/1 -> Sum1/2

== system BrowarModel/Kadz filtracji/Kadz filtracji/Zbiornik dolny/Model jakosci zacieru ==
  note: Model jakosci zacieru
  Objetosc : Inport
  Przepelnienie : Inport  Port=2
  Doplyw zacieru : Inport  Port=3
  Odplyw : Inport  Port=4
  Jakosc zacieru : Inport  Port=5
  Divide1 : Product  Inputs=/*
  Jakosc zacieru x objetosc : Integrator  LimitOutput=on  LowerSaturationLimit=0
  Product3 : Product  RndMeth=Zero
  Product4 : Product  RndMeth=Zero
  Product6 : Product  RndMeth=Zero
  Relational Operator : RelationalOperator  Operator=<  InputSameDT=off
  Sat : Constant
  Sum5 : Sum  Inputs=|+-
  Jakosc zacieru zbiornika : Outport
  wires:
  Sum5/1 -> Jakosc zacieru x objetosc/1
  Product4/1 -> Product3/2
  Sat/1 -> Relational Operator/2
  Jakosc zacieru x objetosc/1 -> Divide1/2
  Divide1/1 -> Product6/1, Jakosc zacieru zbiornika/1
  Product3/1 -> Sum5/1
  Relational Operator/1 -> Product3/1
  Product6/1 -> Sum5/2
  Objetosc/1 -> Divide1/1
  Doplyw zacieru/1 -> Product4/1
  Odplyw/1 -> Product6/2
  Przepelnienie/1 -> Relational Operator/1
  Jakosc zacieru/1 -> Product4/2

== system BrowarModel/Kadz filtracji/Kadz filtracji/Zbiornik dolny/Model utratu ciepla ==
  note: Model utraty ciepla
  Poziom : Inport
  Pole podstawy zbiornika : Inport  Port=2
  Srednia temperatura : Inport  Port=3
  Temperatura lustra : Inport  Port=4
  Cieplo tracone przez pow. gorna : DotProduct  OutDataTypeStr=Inherit: Inherit via internal rule
  Cieplo tracone przez scianki : DotProduct  OutDataTypeStr=Inherit: Inherit via internal rule
  Pow ->obwod : Fcn  Expr=2*3.14*sqrt(u(1)/3.14)
  Pow styku scian bocznych : DotProduct  OutDataTypeStr=Inherit: Inherit via internal rule
  Saturation : Saturate  UpperLimit=inf  LowerLimit=0
  Sum11 : Sum  Inputs=|-+
  Sum12 : Sum  Inputs=|-+
  Sum2 : Sum
  "Temperatura pokojowa (deg C)  " : Constant  Value=22
  Wspolczynnik przenikania ciepla : Gain  Gain=100
  Wspolczynnik przenikania ciepla scian : Gain  Gain=450
  Strumien ciepla : Outport
  wires:
  Saturation/1 -> Strumien ciepla/1  "J/s"
  Wspolczynnik przenikania ciepla/1 -> Cieplo tracone przez pow. gorna/2
  Sum12/1 -> Cieplo tracone przez pow. gorna/1
  Pow ->obwod/1 -> Pow styku scian bocznych/2
  Pow styku scian bocznych/1 -> Wspolczynnik przenikania ciepla scian/1  "m2"
  Wspolczynnik przenikania ciepla scian/1 -> Cieplo tracone przez scianki/1
  Cieplo tracone przez scianki/1 -> Sum2/1
  Cieplo tracone przez pow. gorna/1 -> Sum2/2
  "Temperatura pokojowa (deg C)  "/1 -> Sum11/1, Sum12/1
  Sum11/1 -> Cieplo tracone przez scianki/2
  Poziom/1 -> Pow styku scian bocznych/1
  Pole podstawy zbiornika/1 -> Pow ->obwod/1, Wspolczynnik przenikania ciepla/1
  Srednia temperatura/1 -> Sum11/2  "dec C"
  Sum2/1 -> Saturation/1
  Temperatura lustra/1 -> Sum12/2  "dec C"

== system BrowarModel/Kadz filtracji/Kadz filtracji/Zbiornik dolny/Poziom zbiornik dolny  ==
  note: Poziom zbiornik dolny
  Objetosc : Inport
  Powierzchnia dna : Inport  Port=2
  1/powierzchnia : Product  Inputs=*/
  Pozycja sensora max (3.8 m) : Constant  Value=3.8
  Pozycja sensora min (0.2 m) : Constant  Value=.2
  Sensor max : RelationalOperator  InputSameDT=off
  Sensor min : RelationalOperator  InputSameDT=off
  Poziom  wysoki : Outport
  Poziom niski : Outport  Port=2
  Poziom : Outport  Port=3
  wires:
  Objetosc/1 -> 1/powierzchnia/1
  Powierzchnia dna/1 -> 1/powierzchnia/2
  Sensor min/1 -> Poziom niski/1
  Sensor max/1 -> Poziom  wysoki/1
  Pozycja sensora min (0.2 m)/1 -> Sensor min/2
  Pozycja sensora max (3.8 m)/1 -> Sensor max/2
  1/powierzchnia/1 -> Poziom/1, Sensor max/1, Sensor min/1  "m"

== system BrowarModel/Kadz filtracji/Kadz filtracji/Zbiornik gorny/Model akumulacji ciepla w zbiorniku ==
  note: Model akumulacji ciepla w zbiorniku
  Objetosc cieczy w zbiorniku : Inport
  Przepelnienie : Inport  Port=2
  Strumien odplywu cieczy : Inport  Port=3
  Strumien doplywu wody : Inport  Port=4
  Strumien zacieru : Inport  Port=5
  Temperatura strumien doplywu wody : Inport  Port=6
  Temperatura strumien doplywu zacieru : Inport  Port=7
  Temperatura strumien doplywu brzeczki : Inport  Port=8
  Strumien brzeczki : Inport  Port=9
  Strumien ciepla traconego : Inport  Port=10
  Cieplo : Integrator  InitialCondition=1238534.44  LimitOutput=on  LowerSaturationLimit=0
  Cieplo strumienia cieczy odplywajacej : Subsystem
  Cieplo strumienia doplywajacego : Subsystem
  "Cieplo wlasciwe " : Constant  Value=4189.9
  Divide : Product  Inputs=/*
  Divide1 : Product  Inputs=*/
  Gestosc cieczy : Gain  Gain=1000
  Sum1 : Sum  Inputs=|+-
  Sum3 : Sum  Inputs=|-+
  Sum5 : Sum  Inputs=|+-
  Switch : Switch  Threshold=0.5  SaturateOnIntegerOverflow=off  InputSameDT=off
  Switch1 : Switch  Threshold=-0.5  SaturateOnIntegerOverflow=off  InputSameDT=off
  Zamiana C->K : Constant  Value=273.6
  Zero : Constant  Value=0
  Temperatura : Outport
  wires:
  Strumien odplywu cieczy/1 -> Cieplo strumienia cieczy odplywajacej/2(Strumien cieczy)  "m3/s"
  Gestosc cieczy/1 -> Divide/1  "kg"
  Objetosc cieczy w zbiorniku/1 -> Gestosc cieczy/1  "m3"
  Cieplo/1 -> Divide/2  "J"
  Divide/1 -> Divide1/1
  Divide1/1 -> Cieplo strumienia cieczy odplywajacej/1(Temperatura strumienia cieczy), Sum5/1  "dec K"
  Temperatura strumien doplywu wody/1 -> Cieplo strumienia doplywajacego/1(Temperatura strumienia wody)  "dec C"
  "Cieplo wlasciwe "/1 -> Divide1/2  "J/(kg*K)"
  Zamiana C->K/1 -> Sum5/2
  Strumien doplywu wody/1 -> Cieplo strumienia doplywajacego/2(Strumien wody)  "m3/s"
  Sum5/1 -> Temperatura/1
  Strumien zacieru/1 -> Cieplo strumienia doplywajacego/4(Strumien zacieru)
  Temperatura strumien doplywu zacieru/1 -> Cieplo strumienia doplywajacego/3(Temperatura strumienia zacieru)
  Przepelnienie/1 -> Switch1/2, Switch/2
  Cieplo strumienia doplywajacego/1(Strumien ciepla) -> Switch/3  "J/s"
  Switch/1 -> Sum3/2
  Temperatura strumien doplywu brzeczki/1 -> Cieplo strumienia doplywajacego/5(Temperatura strumienia brzeczki)
  Strumien brzeczki/1 -> Cieplo strumienia doplywajacego/6(Strumien brzeczki)
  Switch1/1 -> Sum3/1
  Cieplo strumienia cieczy odplywajacej/1(Strumien ciepla) -> Switch1/1, Switch/1  "J/s"
  Zero/1 -> Switch1/3
  Sum3/1 -> Sum1/1  "J/s"
  Sum1/1 -> Cieplo/1
  Strumien ciepla traconego/1 -> Sum1/2

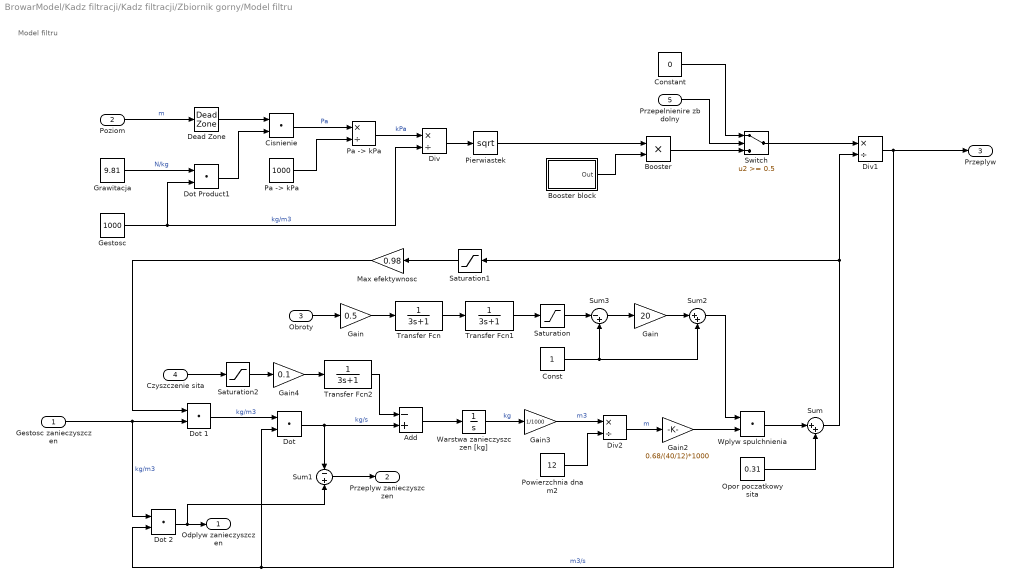
== system BrowarModel/Kadz filtracji/Kadz filtracji/Zbiornik gorny/Model filtru ==
  note: Model filtru
  Gestosc zanieczyszczen : Inport
  Poziom : Inport  Port=2
  Obroty : Inport  Port=3
  Czyszczenie sita : Inport  Port=4
  Przepelnienire zb dolny : Inport  Port=5
  "  Gain " : Gain  Gain=20
  Add : Sum  Inputs=-+
  Booster : Product  RndMeth=Zero
  Booster block : Subsystem
  Cisnienie : DotProduct  OutDataTypeStr=Inherit: Inherit via internal rule
  Const : Constant
  Constant : Constant  Value=0
  Dead Zone : DeadZone  LowerValue=-0.001/12  UpperValue=0.001/12
  Div : Product  Inputs=*/
  Div1 : Product  Inputs=*/
  Div2 : Product  Inputs=*/
  "Dot " : DotProduct  OutDataTypeStr=Inherit: Inherit via internal rule
  Dot 1 : DotProduct  OutDataTypeStr=Inherit: Inherit via internal rule
  Dot 2 : DotProduct  OutDataTypeStr=Inherit: Inherit via internal rule
  Dot Product1 : DotProduct  OutDataTypeStr=Inherit: Inherit via internal rule
  Gain : Gain  Gain=0.5
  Gain2 : Gain  Gain=0.68/(40/12)*1000
  Gain3 : Gain  Gain=1/1000
  Gain4 : Gain  Gain=0.1
  Gestosc : Constant  Value=1000
  Grawitacja : Constant  Value=9.81
  "Max efektywnosc " : Gain  Gain=0.98
  Opor poczatkowy sita : Constant  Value=0.31
  "Pa -> kPa" : Constant  Value=1000
  "Pa -> kPa " : Product  Inputs=*/
  Pierwiastek : Math  Operator=sqrt  SignedPower=on
  "Powierzchnia dna m2 " : Constant  Value=12
  Saturation : Saturate  UpperLimit=1  LowerLimit=0.1
  Saturation1 : Saturate  UpperLimit=1  LowerLimit=0
  Saturation2 : Saturate  UpperLimit=1  LowerLimit=0
  Sum : Sum  Inputs=|++
  Sum1 : Sum  Inputs=-+
  Sum2 : Sum  Inputs=|++
  Sum3 : Sum  Inputs=|-+
  Switch : Switch  Threshold=0.5  SaturateOnIntegerOverflow=off  InputSameDT=off
  Transfer Fcn : TransferFcn  Denominator=[3 1]
  Transfer Fcn1 : TransferFcn  Denominator=[3 1]
  Transfer Fcn2 : TransferFcn  Denominator=[3 1]
  Warstwa zanieczyszczen [kg] : Integrator  LimitOutput=on  LowerSaturationLimit=0
  Wplyw spulchnienia : DotProduct  OutDataTypeStr=Inherit: Inherit via internal rule
  Odplyw zanieczyszczen : Outport
  Przeplyw zanieczyszczen : Outport  Port=2
  Przeplyw : Outport  Port=3
  wires:
  Poziom/1 -> Dead Zone/1  "m"
  Dot Product1/1 -> Cisnienie/2
  Cisnienie/1 -> "Pa -> kPa "/1  "Pa"
  "Pa -> kPa"/1 -> "Pa -> kPa "/2
  Grawitacja/1 -> Dot Product1/1  "N/kg"
  Gestosc/1 -> Dot Product1/2, Div/2  "kg/m3"
  "Pa -> kPa "/1 -> Div/1  "kPa"
  Div/1 -> Pierwiastek/1
  Div1/1 -> "Dot "/2, Dot 2/2, Przeplyw/1  "m3/s"
  "Dot "/1 -> Sum1/1, Add/2  "kg/s"
  Sum/1 -> Div1/2, Saturation1/1
  Opor poczatkowy sita/1 -> Sum/2
  Warstwa zanieczyszczen [kg]/1 -> Gain3/1  "kg"
  Wplyw spulchnienia/1 -> Sum/1
  Transfer Fcn/1 -> Transfer Fcn1/1
  Gain/1 -> Transfer Fcn/1
  Obroty/1 -> Gain/1
  Div2/1 -> Gain2/1  "m"
  "Powierzchnia dna m2 "/1 -> Div2/2
  Dot 2/1 -> Odplyw zanieczyszczen/1, Sum1/2
  Dead Zone/1 -> Cisnienie/1
  Dot 1/1 -> "Dot "/1  "kg/m3"
  Gain3/1 -> Div2/1  "m3"
  "Max efektywnosc "/1 -> Dot 1/1
  Gain2/1 -> Wplyw spulchnienia/2
  Gestosc zanieczyszczen/1 -> Dot 1/2, Dot 2/1  "kg/m3"
  Sum1/1 -> Przeplyw zanieczyszczen/1
  Transfer Fcn1/1 -> Saturation/1
  Sum2/1 -> Wplyw spulchnienia/1
  Const/1 -> Sum2/2, Sum3/2
  "  Gain "/1 -> Sum2/1
  Sum3/1 -> "  Gain "/1
  Saturation/1 -> Sum3/1
  Saturation1/1 -> "Max efektywnosc "/1
  Add/1 -> Warstwa zanieczyszczen [kg]/1
  Czyszczenie sita/1 -> Saturation2/1
  Saturation2/1 -> Gain4/1
  Gain4/1 -> Transfer Fcn2/1
  Transfer Fcn2/1 -> Add/1
  Pierwiastek/1 -> Booster/1
  Booster block/1(Out) -> Booster/2
  Booster/1 -> Switch/3
  Switch/1 -> Div1/1
  Przepelnienire zb dolny/1 -> Switch/2
  Constant/1 -> Switch/1

== system BrowarModel/Kadz filtracji/Kadz filtracji/Zbiornik gorny/Model jakosci zacieru ==
  note: Model jakosci zacieru
  Odplyw : Inport
  Objetosc : Inport  Port=2
  Przepelnienie : Inport  Port=3
  Doplyw zacieru : Inport  Port=4
  Doplyw brzeczki : Inport  Port=5
  Jakosc zacieru : Inport  Port=6
  Jakosc zacieru brzeczki : Inport  Port=7
  Divide1 : Product  Inputs=/*
  Jakosc zacieru x objetosc : Integrator  LimitOutput=on  LowerSaturationLimit=0
  Product{3..6} (4 alike) : Product  RndMeth=Zero
  Relational Operator : RelationalOperator  Operator=<  InputSameDT=off
  Sat : Constant
  Sum5 : Sum  Inputs=|+-
  Sum6 : Sum  Inputs=|++
  Jakosc zacieru zbiornika : Outport
  wires:
  Sum5/1 -> Jakosc zacieru x objetosc/1
  Product4/1 -> Sum6/1
  Sat/1 -> Relational Operator/2
  Jakosc zacieru x objetosc/1 -> Divide1/2
  Divide1/1 -> Product6/1, Jakosc zacieru zbiornika/1
  Product3/1 -> Sum5/1
  Relational Operator/1 -> Product3/1
  Sum6/1 -> Product3/2
  Product5/1 -> Sum6/2
  Product6/1 -> Sum5/2
  Objetosc/1 -> Divide1/1
  Doplyw zacieru/1 -> Product4/1
  Odplyw/1 -> Product6/2
  Przepelnienie/1 -> Relational Operator/1
  Jakosc zacieru/1 -> Product4/2
  Jakosc zacieru brzeczki/1 -> Product5/2
  Doplyw brzeczki/1 -> Product5/1

== system BrowarModel/Kadz filtracji/Kadz filtracji/Zbiornik gorny/Model masy zanieczyszczen ==
  note: Model masy zanieczyszczen
  Odplyw zanieczyszczen : Inport
  Gestosc zanieczyszczen brzeczki przedniej : Inport  Port=2
  Doplyw wody : Inport  Port=3
  Doplyw zacieru : Inport  Port=4
  Doplyw brzeczki przedniej : Inport  Port=5
  Brzeczka przednia : DotProduct  OutDataTypeStr=Inherit: Inherit via internal rule
  Gestosc zanieczyszczen woda : Constant  Value=0
  Gestosc zanieczyszczen zacier : Constant  Value=1.1
  "Masa zanieczyszczen " : Integrator  InitialCondition=0.001*1.1  LimitOutput=on  LowerSaturationLimit=0.001*1.1
  Sum1 : Sum  Inputs=+++
  Sum2 : Sum  Inputs=|+-
  Woda : DotProduct  OutDataTypeStr=Inherit: Inherit via internal rule
  Zacier : DotProduct  OutDataTypeStr=Inherit: Inherit via internal rule
  Masa zanieczyszczen : Outport
  wires:
  Woda/1 -> Sum1/1  "kg/s"
  Zacier/1 -> Sum1/2  "kg/s"
  Brzeczka przednia/1 -> Sum1/3  "kg/s"
  Gestosc zanieczyszczen zacier/1 -> Zacier/1  "kg/m3"
  Gestosc zanieczyszczen woda/1 -> Woda/1  "kg/m3"
  Doplyw wody/1 -> Woda/2  "m3/s"
  Doplyw zacieru/1 -> Zacier/2  "m3/s"
  Doplyw brzeczki przedniej/1 -> Brzeczka przednia/2  "m3/s"
  "Masa zanieczyszczen "/1 -> Masa zanieczyszczen/1  "kg"
  Gestosc zanieczyszczen brzeczki przedniej/1 -> Brzeczka przednia/1  "kg/m3"
  Sum1/1 -> Sum2/1  "kg/s"
  Sum2/1 -> "Masa zanieczyszczen "/1  "kg/s"
  Odplyw zanieczyszczen/1 -> Sum2/2  "kg/s"

== system BrowarModel/Kadz filtracji/Kadz filtracji/Zbiornik gorny/Model mieszadla ==
  note: Model mieszadla
  Obroty : Inport
  Poslizg przekladni : Inport  Port=2
  " Gain" : Gain  Gain=1/4
  " Gain1" : Gain  Gain=1/100
  " Redukcja obrotow" : Gain  Gain=2/1440
  Constant : Constant  Value=100
  Dot : DotProduct  OutDataTypeStr=Inherit: Inherit via internal rule
  Math Function : Math  Operator=square  SignedPower=on
  Sat FS : Saturate  UpperLimit=1  LowerLimit=0
  Sat uszkodzenia [0,100] : Saturate  UpperLimit=100  LowerLimit=0
  Sum1 : Sum  Inputs=|-+
  Obroty zredukowane : Outport
  Obciazenie : Outport  Port=2
  wires:
  Sat FS/1 -> Obciazenie/1
  " Gain"/1 -> Sat FS/1
  Math Function/1 -> " Gain"/1
  Obroty/1 -> " Redukcja obrotow"/1  "obr/min"
  Poslizg przekladni/1 -> Sat uszkodzenia [0,100]/1  "[0,100]"
  Sat uszkodzenia [0,100]/1 -> Sum1/1
  Sum1/1 -> " Gain1"/1
  Constant/1 -> Sum1/2
  " Redukcja obrotow"/1 -> Dot/2  "obr/min"
  Dot/1 -> Obroty zredukowane/1, Math Function/1
  " Gain1"/1 -> Dot/1

== system BrowarModel/Kadz filtracji/Kadz filtracji/Zbiornik gorny/Model utratu ciepla ==
  note: Model utraty ciepla
  Poziom : Inport
  Pole podstawy zbiornika : Inport  Port=2
  Srednia temperatura : Inport  Port=3
  Temperatura lustra : Inport  Port=4
  Cieplo tracone przez pow. gorna : DotProduct  OutDataTypeStr=Inherit: Inherit via internal rule
  Cieplo tracone przez scianki : DotProduct  OutDataTypeStr=Inherit: Inherit via internal rule
  Pow ->obwod : Fcn  Expr=2*3.14*sqrt(u(1)/3.14)
  Pow styku scian bocznych : DotProduct  OutDataTypeStr=Inherit: Inherit via internal rule
  Saturation : Saturate  UpperLimit=inf  LowerLimit=0
  Sum11 : Sum  Inputs=|-+
  Sum12 : Sum  Inputs=|-+
  Sum2 : Sum
  "Temperatura pokojowa (deg C)  " : Constant  Value=22
  Wspolczynnik przenikania ciepla : Gain  Gain=450
  Wspolczynnik przenikania ciepla scian : Gain  Gain=450
  Strumien ciepla : Outport
  wires:
  Saturation/1 -> Strumien ciepla/1  "J/s"
  Wspolczynnik przenikania ciepla/1 -> Cieplo tracone przez pow. gorna/2
  Sum12/1 -> Cieplo tracone przez pow. gorna/1
  Pow ->obwod/1 -> Pow styku scian bocznych/2
  Pow styku scian bocznych/1 -> Wspolczynnik przenikania ciepla scian/1  "m2"
  Wspolczynnik przenikania ciepla scian/1 -> Cieplo tracone przez scianki/1
  Cieplo tracone przez scianki/1 -> Sum2/1
  Cieplo tracone przez pow. gorna/1 -> Sum2/2
  "Temperatura pokojowa (deg C)  "/1 -> Sum11/1, Sum12/1
  Sum11/1 -> Cieplo tracone przez scianki/2
  Poziom/1 -> Pow styku scian bocznych/1
  Pole podstawy zbiornika/1 -> Pow ->obwod/1, Wspolczynnik przenikania ciepla/1
  Srednia temperatura/1 -> Sum11/2  "dec C"
  Sum2/1 -> Saturation/1
  Temperatura lustra/1 -> Sum12/2  "dec C"

== system BrowarModel/Kadz filtracji/Kadz filtracji/Zbiornik gorny/Poziom zbiornik gorny  ==
  note: Poziom zbiornik gorny
  Objetosc : Inport
  Powierzchnia dna : Inport  Port=2
  1/powierzchnia : Product  Inputs=*/
  Pozycja sensora max (1.8 m) : Constant  Value=1.8
  Pozycja sensora min (0.2 m) : Constant  Value=.2
  Sensor max : RelationalOperator  InputSameDT=off
  Sensor min : RelationalOperator  InputSameDT=off
  Poziom  wysoki : Outport
  Poziom niski : Outport  Port=2
  Poziom : Outport  Port=3
  wires:
  1/powierzchnia/1 -> Sensor min/1, Sensor max/1, Poziom/1  "m"
  Pozycja sensora max (1.8 m)/1 -> Sensor max/2
  Pozycja sensora min (0.2 m)/1 -> Sensor min/2
  Sensor max/1 -> Poziom  wysoki/1
  Sensor min/1 -> Poziom niski/1
  Powierzchnia dna/1 -> 1/powierzchnia/2
  Objetosc/1 -> 1/powierzchnia/1
